simulink subsystem "Outputs_ESP32"  (R2023b)
settings: Solver=VariableStepAuto  StartTime=0.0  StopTime=10.0  RelTol=1e-3
libraries: arduinolib x9
settings Model: Creator=m4ttn  LastModifiedBy=m4ttn
settings RTWCC: GPUComputeCapability=5.0

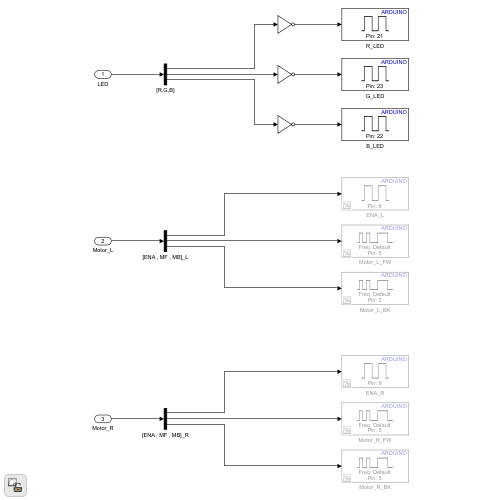
[thumbnail: Simulink's stored preview of the top-level diagram]
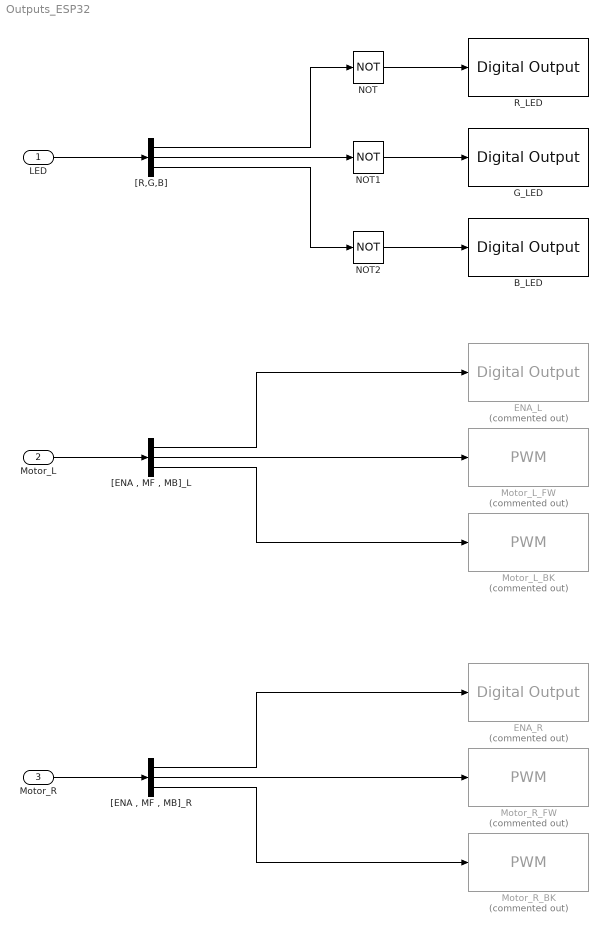
== system Outputs_ESP32 ==
  LED : Inport
  Motor_L : Inport  Port=2
  Motor_R : Inport  Port=3
  B_LED : arduinolib/Digital Output  pinNumber=22  Direction=output  blockPlatform=arduino
  ENA_L : arduinolib/Digital Output  Commented=on  pinNumber=9  Direction=output  blockPlatform=arduino
  ENA_R : arduinolib/Digital Output  Commented=on  pinNumber=9  Direction=output  blockPlatform=arduino
  G_LED : arduinolib/Digital Output  pinNumber=23  Direction=output  blockPlatform=arduino
  Motor_L_BK : arduinolib/PWM  Commented=on  pinNumber=5  frequencyType=Default  desiredFrequency=490.2  achievableFrequency=490.2
  Motor_L_FW : arduinolib/PWM  Commented=on  pinNumber=5  frequencyType=Default  desiredFrequency=490.2  achievableFrequency=490.2
  Motor_R_BK : arduinolib/PWM  Commented=on  pinNumber=5  frequencyType=Default  desiredFrequency=490.2  achievableFrequency=490.2
  Motor_R_FW : arduinolib/PWM  Commented=on  pinNumber=5  frequencyType=Default  desiredFrequency=490.2  achievableFrequency=490.2
  NOT : Logic  Operator=NOT  IconShape=distinctive  AllPortsSameDT=off  OutDataTypeStr=boolean
  NOT1 : Logic  Operator=NOT  IconShape=distinctive  AllPortsSameDT=off  OutDataTypeStr=boolean
  NOT2 : Logic  Operator=NOT  IconShape=distinctive  AllPortsSameDT=off  OutDataTypeStr=boolean
  R_LED : arduinolib/Digital Output  pinNumber=21  Direction=output  blockPlatform=arduino
  "[ENA , MF , MB]_L" : Demux  Outputs=3
  "[ENA , MF , MB]_R" : Demux  Outputs=3
  "[R,G,B]" : Demux  Outputs=3
  wires:
  LED/1 -> "[R,G,B]"/1
  "[R,G,B]"/1 -> NOT/1
  "[R,G,B]"/2 -> NOT1/1
  "[R,G,B]"/3 -> NOT2/1
  Motor_L/1 -> "[ENA , MF , MB]_L"/1
  "[ENA , MF , MB]_L"/1 -> ENA_L/1
  "[ENA , MF , MB]_L"/2 -> Motor_L_FW/1
  "[ENA , MF , MB]_L"/3 -> Motor_L_BK/1
  Motor_R/1 -> "[ENA , MF , MB]_R"/1
  "[ENA , MF , MB]_R"/3 -> Motor_R_BK/1
  "[ENA , MF , MB]_R"/1 -> ENA_R/1
  "[ENA , MF , MB]_R"/2 -> Motor_R_FW/1
  NOT/1 -> R_LED/1
  NOT1/1 -> G_LED/1
  NOT2/1 -> B_LED/1
